simulink model "me132LabPartF"  (R2021a)
settings: Solver=VariableStepAuto  StartTime=0.0  StopTime=10.0  RelTol=1e-3
settings Model: Creator=kaiyu  LastModifiedBy=kaiyu

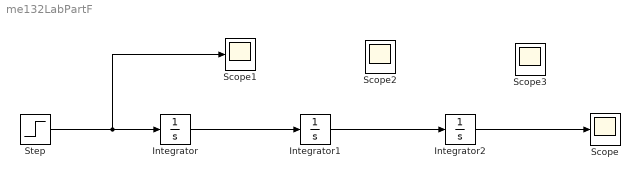
== system me132LabPartF ==
  Integrator : Integrator
  Integrator1 : Integrator
  Integrator2 : Integrator
  Scope : Scope
  Scope1 : Scope
  Scope2 : Scope  NumInputPorts=2
  Scope3 : Scope
  Step : Step  SampleTime=0
  wires:
  Step/1 -> Scope1/1, Integrator/1
  Integrator/1 -> Integrator1/1
  Integrator1/1 -> Integrator2/1
  Integrator2/1 -> Scope/1
